simulink model "pumps"  (R2013a)
settings: Solver=ode45  StartTime=0.0  StopTime=10.0  RelTol=1e-3
undefined symbols (not defined in the file or in its folder): Dmax, n_mech, p_nom, rho_nom, v_nom, wp_nom, xp_max
settings Model: Creator=Toshiba  LastModifiedBy=Toshiba

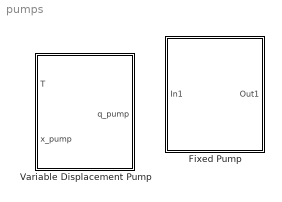
== system pumps ==
  Fixed Pump : Subsystem
  Variable Displacement Pump : Subsystem

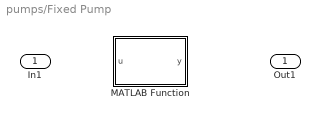
== system pumps/Fixed Pump ==
  In1 : Inport
  MATLAB Function : MATLAB Function  TreatAsAtomicUnit=on
  Out1 : Outport

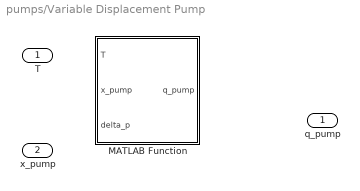
== system pumps/Variable Displacement Pump ==
  T : Inport
  x_pump : Inport  Port=2
  MATLAB Function : MATLAB Function  TreatAsAtomicUnit=on
  q_pump : Outport

== matlab function pumps/Fixed Pump/MATLAB Function ==
  data: u input; y output
function y = fcn(u)
%#codegen

y = u;

== matlab function pumps/Variable Displacement Pump/MATLAB Function ==
  data: T input; q_pump output; x_pump input; delta_p input; Dmax parameter; xp_max parameter; wp_nom parameter; v_nom parameter; rho_nom parameter; p_nom parameter; n_mech parameter
function q_pump = fcn(T,x_pump,delta_p, Dmax,xp_max,wp_nom,v_nom,rho_nom,p_nom, n_mech)
%#codegen

D = Dmax*x_pump / xp_max;
Kleak = Khp / (v*rho);


q_pump = D*w - Kleak*delta_p;
